simulink model "teamduo"  (R2024b)
settings: Solver=FixedStepAuto  StartTime=0.0  StopTime=10.0  RelTol=1e-3
libraries: robotlib x5
settings Model: Creator=max  LastModifiedBy=jasonmok
settings OptimizationCC: EnhancedBackFolding=on  PassReuseOutputArgsThreshold=0  MaxStackSize=64  OptimizeBlockOrder=speed  DifferentSizesBufferReuse=on  OptimizationCustomize=off
settings DebuggingCC: ParameterTunabilityLossMsg=error
settings HardwareCC: ProdBitPerPointer=32  ProdBitPerSizeT=32  ProdBitPerPtrDiffT=32  ProdLargestAtomicFloat=None  ProdIntDivRoundTo=Undefined  ProdEndianess=Unspecified  ProdWordSize=32  ProdHWDeviceType=Generic->Unspecified (assume 32-bit Generic)  UseEmbeddedCoderFeatures=off
settings SFSimCC: MATLABDynamicMemAlloc=off
settings RTWCC: Description=Embedded Coder  SystemTargetFile=ert.tlc  HardwareBoard=Robot Operating System (ROS)  TLCOptions="-aInlineSetEventsForThisBaseRateFcn=TLC_FALSE -aSuppressMultiTaskScheduler=TLC_FALSE  -aRateBasedStepFcn=0"  TemplateMakefile=ert_default_tmf  Toolchain=Catkin  TargetLang=C++
settings CodeAppCC: ForceParamTrailComments=on  OperatorAnnotations=on
settings ERTTargetCC: ERTCustomFileBanners=off  SupportContinuousTime=on  SupportNonInlinedSFcns=on  RemoveResetFunc=off  ModelStepFunctionPrototypeControlCompliant=off  InlinedParameterPlacement=Hierarchical  DynamicArrayContainerType=coder::array

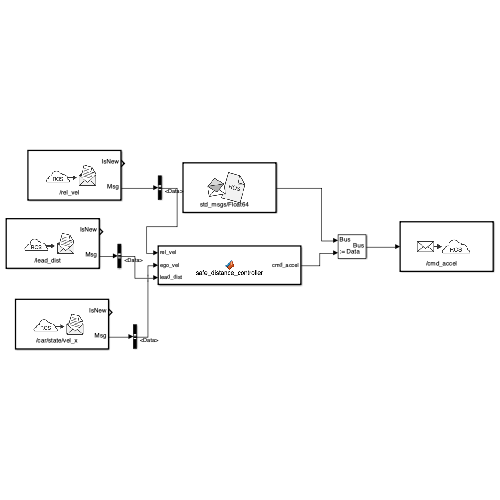
[thumbnail: Simulink's stored preview of the top-level diagram]
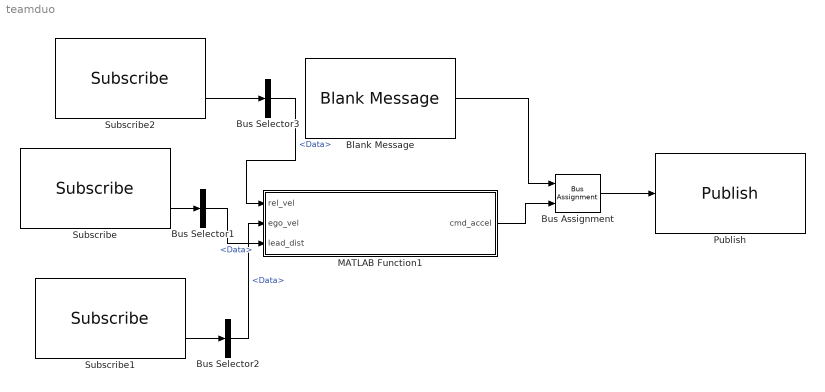
== system teamduo ==
  Blank Message : robotlib/Blank Message  messageClass=Message  entityType=std_msgs/Float64  messageType=std_msgs/Float64  SampleTime=inf  legacyBusStruct=off
  Bus Assignment : BusAssignment  AssignedSignals=Data
  Bus Selector1 : BusSelector  OutputSignals=Data
  Bus Selector2 : BusSelector  OutputSignals=Data
  Bus Selector3 : BusSelector  OutputSignals=Data
  MATLAB Function1 : MATLAB Function  TreatAsAtomicUnit=on
  Publish : robotlib/Publish  topicSource=Specify your own  topic=/cmd_accel  messageType=std_msgs/Float64  legacyBusStruct=off  messageQueueLength=1
  Subscribe : robotlib/Subscribe  topicSource=Specify your own  topic=/lead_dist  messageType=std_msgs/Float64  SampleTime=-1  legacyBusStruct=off  messageQueueLength=1
  Subscribe1 : robotlib/Subscribe  topicSource=Specify your own  topic=/car/state/vel_x  messageType=std_msgs/Float64  SampleTime=-1  legacyBusStruct=off  messageQueueLength=1
  Subscribe2 : robotlib/Subscribe  topicSource=Specify your own  topic=/rel_vel  messageType=std_msgs/Float64  SampleTime=-1  legacyBusStruct=off  messageQueueLength=1
  wires:
  Subscribe/2 -> Bus Selector1/1
  Subscribe1/2 -> Bus Selector2/1
  MATLAB Function1/1(cmd_accel) -> Bus Assignment/2
  Blank Message/1 -> Bus Assignment/1
  Bus Selector2/1 -> MATLAB Function1/2(ego_vel)  "<Data>"
  Bus Assignment/1 -> Publish/1
  Bus Selector1/1 -> MATLAB Function1/3(lead_dist)  "<Data>"
  Subscribe2/2 -> Bus Selector3/1
  Bus Selector3/1 -> MATLAB Function1/1(rel_vel)  "<Data>"

== matlab function teamduo/MATLAB Function1 ==
  data: rel_vel input; cmd_accel output; ego_vel input; lead_dist input
function cmd_accel = safe_distance_controller(rel_vel, ego_vel, lead_dist)
    % Parameters
    tau = 3; % Desired time gap in seconds
    alpha = 1; % Gain factor for time gap control
    beta = 2; % Gain factor for relative velocity compensation
    max_accel = 3; % Maximum allowable acceleration (m/s^2)
    min_accel = -3; % Minimum allowable deceleration (m/s^2)
    
    % Calculate the desired safe distance based on the time gap
    safe_distance = tau * ego_vel;
    
    % Calculate the distance error
    distance_error = lead_dist - safe_distance;
    
    % Control law: combine distance control and relative velocity compensation
    cmd_accel = alpha * distance_error + beta * (-rel_vel);
    
    % Cap the acceleration to within the allowable range
    if cmd_accel > max_accel
        cmd_accel = max_accel;
    elseif cmd_accel < min_accel
        cmd_accel = min_accel;
    end
end
